simulink subsystem "PvtSubSys_LATC"  (R2020b)
settings: Solver=VariableStepAuto  StartTime=0.0  StopTime=10.0  RelTol=1e-3
undefined symbols (not defined in the file or in its folder): LCS_PLAN_PreViewIdxNum, LCS_PLAN_PreViewIdxSW_b, P_Global_CharSpd_ms, P_Global_SteeringAngleRatio, P_Global_WheelBase_m, P_LCS_DetNoOverRide_DrvTrq_TH, P_LCS_DetOverRide_DrvTrq_TH, P_LCS_ESS_AngleSlope_Limit, P_LCS_ESS_LogicTest_Enable, P_LCS_ESS_NotActiveFlgDelayTime, P_LCS_ESS_NotActiveFlgDelayTimeSW, P_LCS_ESS_SteerAngleErr, P_LCS_ESS_SteerAngleFilterTime, P_LCS_ESS_TarAngleFilterTime, P_LCS_ESSAngleSW, P_LCS_ESSOverrideTime1, P_LCS_ESSOverrideTime2, P_LCS_ESSOverrideTime3, P_LCS_ESSOverrideValue1, P_LCS_ESSOverrideValue2, P_LCS_IN_Offset_Test_SW, P_LCS_IN_Offset_Test_Value, P_LCS_LATC_AngleFilterTime_s, P_LCS_LATC_CurOffsetA2FliterT_s, P_LCS_LATC_CurOffsetCurve_TabX_m, P_LCS_LATC_CurOffsetCurveFliterTime_Tab_s, P_LCS_LATC_CurOffsetVehicleSpdLimitValue_degs, P_LCS_LATC_DeltaEps_Tab_s, P_LCS_LATC_DxOffset_Sw, P_LCS_LATC_ELKAngleSlope_ratio, P_LCS_LATC_ELKMaxLatAcc_ms2, P_LCS_LATC_ESSA0Dis_TabX_m, P_LCS_LATC_ESSAddAngleSlope_Tab_degs, P_LCS_LATC_ESSAESAngleSlope_Tab_degs, P_LCS_LATC_ESSAngleSlope_ratio, P_LCS_LATC_ESSMaxLatAcc_ms2, P_LCS_LATC_LCAngleSlope_ratio, P_LCS_LATC_LCAngleSlope_Tab_degs, P_LCS_LATC_LCCancleMaxLatAcc_ms2, P_LCS_LATC_LCEcoAngleSlope_ratio, P_LCS_LATC_LCEcoAngleSlope_Tab_degs, P_LCS_LATC_LCEcoMaxLatAcc_ms2, P_LCS_LATC_LCKAngleSlope_ratio, P_LCS_LATC_LCKAngleSlope_Tab_degs, P_LCS_LATC_LCKIEAngleSlope_ratio, P_LCS_LATC_LCKIEAngleSlope_Tab_degs, P_LCS_LATC_LCKIEMaxLatAcc_ms2, P_LCS_LATC_LCKMaxLatAcc_ms2, P_LCS_LATC_LCNormalAngleSlope_ratio, P_LCS_LATC_LCNormalAngleSlope_Tab_degs, P_LCS_LATC_LCNormalMaxLatAcc_ms2, P_LCS_LATC_LCSportAngleSlope_ratio, P_LCS_LATC_LCSportAngleSlope_Tab_degs, P_LCS_LATC_LCSportMaxLatAcc_ms2, P_LCS_LATC_LKAAngleSlope_ratio, P_LCS_LATC_LKAAngleSlope_Tab_degs, P_LCS_LATC_LKAMaxLatAcc_ms2, P_LCS_LATC_MatrixQ1_st, P_LCS_LATC_MatrixQ3_st, P_LCS_LATC_MatrixR_st ... (+71)
libraries: simulink x38
(part 6 of 6)

== matlab function PvtSubSys_LATC/LATC/LateralControl/LCS_Angle/Lateral_Control/kinematics_MPC/SteerAngSlopeCalc/MATLAB Function3 ==
  data: delytime input uint16; TarDangerLevel input uint8; TarDangerLevelK1 input uint8; FLg output uint8; FLgK1 input uint8; CntK1 input uint16; Cnt output uint16
function [FLg,Cnt] = AngSlopeCalc(delytime,TarDangerLevel,TarDangerLevelK1,FLgK1,CntK1)

Cnt = min(CntK1 + uint16(1),delytime);
if Cnt== delytime
    FLg = uint8(0);
else
    FLg = FLgK1;
end
%FLg = FLgK1;
%% 
if TarDangerLevel==uint8(1) && TarDangerLevelK1==0  % NO function 2 LCK (TarDangerLevelK1==0)
    Cnt =uint16(0);
    FLg = uint8(1);
end

if  TarDangerLevel==uint8(3) && (TarDangerLevelK1==uint8(1)||TarDangerLevelK1==uint8(2)) % LCK/IE 2 LC_Normal
    Cnt =uint16(0);
    FLg = uint8(2);
end

if  TarDangerLevel==uint8(7) && (TarDangerLevelK1==uint8(1)||TarDangerLevelK1==uint8(2)) % LCK/IE 2 LC_Eco
    Cnt =uint16(0);
    FLg = uint8(3);
end

if  TarDangerLevel==uint8(8) && (TarDangerLevelK1==uint8(1)||TarDangerLevelK1==uint8(2)) % LCK/IE 2 LC_sport
    Cnt =uint16(0);
    FLg = uint8(4);
end
if  TarDangerLevel==uint8(6) && (TarDangerLevelK1==uint8(1)||TarDangerLevelK1==uint8(2)) % LCK/IE 2 ESS 后期添加配和ESS Slope 一起调试
    Cnt =uint16(0);
    FLg = uint8(5);
end

== matlab function PvtSubSys_LATC/LATC/LateralControl/LCS_Angle/Lateral_Control/kinematics_MPC/TarSteerAngleCalc ==
  data: steer_angle_cmd_temp output; steer_feedforward_temp output; steer_feedbackward_temp output; steer_limit_temp output; matrix_result output; LineValid input; SteerAngle input; steer_angle output size=[1,1]; Veh_Speed input; ref_curve input; ref_theta input; Delta_t input; lateral_error input; heading_error input; Umax input; Delta_umax input; Left_steer_ratio input; Right_steer_ratio input; Matrix_q1 input; Matrix_q2 input; Matrix_r input; Max_lateral_acceleration input; TarSteerAngleSlope input; CurrentSteerAngleOffset input; steer_angleK1 input single; U_k output; U_k1 input single
function [steer_angle_cmd_temp,steer_feedforward_temp,steer_feedbackward_temp,steer_limit_temp,matrix_result,steer_angle,U_k]= ...
    kinematics_MPC(LineValid,SteerAngle,Veh_Speed,ref_curve,ref_theta,Delta_t,lateral_error,heading_error,Umax,Delta_umax,...
    Left_steer_ratio,Right_steer_ratio,Matrix_q1,Matrix_q2,Matrix_r,Max_lateral_acceleration,TarSteerAngleSlope,CurrentSteerAngleOffset,steer_angleK1,U_k1)
if LineValid
    %% 1.车辆参数
    %1.1 车的大小及长度参数
    veh_params.vehicle_length = single(4.875);
    veh_params.vehicle_width  = single(2.2);
    veh_params.vehicle_height = single(1.69);
    %1.2 车辆控制参数
    veh_params.wheel_base = single(2.92);               %轴距, m
    veh_params.Vch = single(23.5);                      %特征车速
    veh_params.max_steer_angle = single(53 / 180 * pi); %前轮最大转角  
    veh_params.max_acceleration = single(2);            %车辆最大加速度
    veh_params.max_deceleration = single(-2);           %车辆最大减速度
    veh_params.left_steer_ratio = Left_steer_ratio;     %车辆左侧转向传动比%
    veh_params.right_steer_ratio = Right_steer_ratio;   %车辆右侧转向传动比%
    veh_params.cf = single(155494.663);                 %车辆前轮侧偏刚度
    veh_params.cr = single(155494.663);                 %车辆后轮侧偏刚度 
    veh_params.mass_fl = single(520);                   %车辆左前轮负重
    veh_params.mass_fr = single(520);                   %车辆右前轮负重
    veh_params.mass_rl = single(520);                   %车辆左后轮负重
    veh_params.mass_rr = single(520);                   %车辆右后轮负重
    %% 2.控制参数计算
    %% 3.MPC矩阵
    Np = single(10);
    Nc = single(5);
    Row = single(10); %松弛因子
    ref_delta = atan(veh_params.wheel_base * ref_curve);   %前轮转角
    
    A = [ 1  Veh_Speed * cos(ref_theta) * Delta_t;
          0  1 ];
    B = [ 0;
        Veh_Speed * Delta_t / (veh_params.wheel_base * cos(ref_delta)^2)];
    Nx = size(A,1); %状态量的个数 2
    Nu = size(B,2); %控制量的个数 1
    % 对状态量进行增广
    kesi = zeros(Nx,1); % 构造新的状态量矩阵
    kesi = cat(1,kesi,U_k1);% 将上一时刻的前轮偏角误差放在第3行，进行状态增广3*1维矩阵
    kesi(1) = lateral_error;
    kesi(2) = heading_error;
    %定义Q和R矩阵
    matrix_q = [Matrix_q1 0;
                0 Matrix_q2];
    matrix_r = Matrix_r;
    matrix_Q = zeros(Np*Nx,Np*Nx);%20*20
    matrix_Q_temp = zeros(Nx,Np*Nx);%2*20
    for i=1:Np
        for j= 1:Np
            if i == j
                matrix_Q_temp = zeros(Nx,Np*Nx);
                matrix_Q_temp(:,((j-1)*Nx+1):j*Nx) = matrix_q;
            end
        end
        matrix_Q(((i-1)*Nx+1):i*Nx,:) = matrix_Q_temp;
    end
    matrix_R = zeros(Nc*Nu,Nc*Nu);%10*10
    matrix_R_temp = zeros(Nu,Nc*Nu);
    for i=1:Nc
        for j= 1:Nc
            if i == j
                matrix_R_temp = zeros(Nu,Nc*Nu);
                matrix_R_temp(:,((j-1)*Nu+1):j*Nu) = matrix_r;
            end
        end
        matrix_R(((i-1)*Nu+1):i*Nu,:) = matrix_R_temp;
    end
    % 按增量式对矩阵进行增广
    A = [A B;zeros(Nu,Nx) eye(Nu)]; % 3*3
    B = [B;eye(Nu)]; % 3*1
    % 定义输出矩阵
    C = single([1 0 0;0 1 0;]);% 2*3
    % THETA和PHI
    PHI = zeros(Np*Nx,size(A,2));
    THETA = zeros(Np*Nx,Nc*Nu);
    THETA_temp = zeros(Nx,Nc*Nu);
    for r=1:Np
        for c=1:Nc
            if c<=r
                THETA_temp(:,((c-1)*Nu+1):c*Nu)=C*A^(r-c)*B; %2*3*3*3*1
            end
        end
        THETA(((r-1)*Nx+1):r*Nx,:) = THETA_temp;
        PHI(((r-1)*Nx+1):r*Nx,:) =  C*A^r; %2*3*3*3
    end
    
    % 构造二次规划的H矩阵
    H_temp = THETA'*matrix_Q*THETA + matrix_R;
    % H = zeros((size(H_temp,1)+1),(size(H_temp,2)+1));
    H = [H_temp zeros(Nu*Nc,1);zeros(1,Nu*Nc) Row];
    H = single(2)*H;
    H = (H+H')/single(2);
    % E矩阵
    error = PHI*kesi; %这里的error就是我们所设的E矩阵
    % f矩阵
    f_temp = single(2)*error'* matrix_Q * THETA;
    f = zeros(size(f_temp,1),(size(f_temp,2)+1));
    f(:,1:size(f_temp,2)) = f_temp;
    %% 约束生成区域
    % 不等式约束
    A_t = tril(ones(Nc,Nc),0);
    A_I=kron(A_t,eye(Nu));
    Ut=kron(ones(Nc,1),U_k1);                 %此处的U表示的应该是上一时刻控制量误差（即偏差）组成的矩阵。
    umin = -Umax/single(57.3);                %维数与控制变量的个数相同
    umax = Umax/single(57.3);                 %此处的最大值最小值约束，是对控制量误差的最大最小值进行约束，此处理解的物理意义是在参考转角上下一个范围内进行约束求解
    
    delta_umin =  -Delta_umax/single(57.3)*Delta_t;
    delta_umax =   Delta_umax/single(57.3)*Delta_t;
    Umin=kron(ones(Nc,1),umin);
    Umax=kron(ones(Nc,1),umax);
%     A_cons = [A_I zeros(Nu*Nc,1);-A_I zeros(Nu*Nc,1)];
%     b_cons = [Umax-Ut;-Umin+Ut];
    % 上下限约束
    EM = single(10);
    delta_Umin=kron(ones(Nc,1),delta_umin);
    delta_Umax=kron(ones(Nc,1),delta_umax);
    lb=[delta_Umin;-EM];%（求解方程）状态量下界，包含控制时域内控制增量和松弛因子下界M
    ub=[delta_Umax;EM];%（求解方程）状态量上界，包含控制时域内控制增量和松弛因子上界M
    % 两种约束合并
    A_cons2 = [A_I zeros(Nu*Nc,1);-A_I zeros(Nu*Nc,1);eye((Nu*Nc)+1);-eye((Nu*Nc)+1)];
    b_cons2 = [Umax-Ut;-Umin+Ut;ub;-lb];
    %% 二次规划求解
    % Format in qp_solver
    % min 0.5*x'*H*x + f'*x   subject to:  A*x <= b
    % with respect to:  A * x = b (equality constraint)
    % A*x <= b (inequality constraint)
    % solve QR problem
    % [matrix_result] = mpcCustomSolverCodeGen(single(H),single(f), single(-A_cons2), single(-b_cons2));
    matrix_result = single(zeros(Nc+1,1));
    matrix_result = MPC_Solver_QPhild(H,f',A_cons2,b_cons2);
    %% 4.计算前轮转角
    u_piao = matrix_result(1);
    U_k = single(kesi(3)) + u_piao;
    steer_cmd = ref_delta + U_k;
    %% 反算方向盘转角并转换为角度制
    if (steer_cmd>=0)
        steer_transmission_ratio = veh_params.left_steer_ratio;
    else
        steer_transmission_ratio = veh_params.right_steer_ratio;
    end
    steer_feedforward_temp  = ref_delta * single(57.3) * steer_transmission_ratio;%反算方向盘转角并转换为角度制deg
    steer_feedbackward_temp = U_k * single(57.3) * steer_transmission_ratio;%反算方向盘转角并转换为角度制deg
    steer_angle_cmd = steer_cmd * single(57.3) * steer_transmission_ratio;%反算方向盘转角并转换为角度制deg
    steer_angle_cmd_temp = steer_angle_cmd;%输出算法计算角度作为观测，最终请求角度会补偿转向不足。
    %% 5.限制期望前轮偏角
    % 5.1 根据横向加速度限制前轮转角
    if Veh_Speed < 1
        steer_limit = atan( Max_lateral_acceleration * veh_params.wheel_base /(Veh_Speed *Veh_Speed))* single(57.3) * steer_transmission_ratio; % 高速计算不准确，更改为下面特征车速计算方法
    else
        AckConst = min((single(1)+Veh_Speed*Veh_Speed/(veh_params.Vch*veh_params.Vch))*veh_params.wheel_base/max(single(1),Veh_Speed),single(32767));
        % PsiDtAckRaw = (SteerAngle/steer_transmission_ratio)/AckConst;
        steer_limit = ((Max_lateral_acceleration * AckConst)/Veh_Speed)* single(57.3) * steer_transmission_ratio;
    end
    %     steer_limit = atan( Max_lateral_acceleration * veh_params.wheel_base /(Veh_Speed *Veh_Speed)) * steer_transmission_ratio;
    steer_angle_cmd = min(steer_limit, max(-steer_limit,steer_angle_cmd));%方向盘角度制deg
    
    steer_angle_deg = steer_angle_cmd + CurrentSteerAngleOffset;
    steer_limit_temp = steer_limit;
    % 5.2 限制方向盘转速
    steer_angle = min(steer_angleK1 + TarSteerAngleSlope,max(steer_angleK1 - TarSteerAngleSlope,steer_angle_deg));
    
else
    U_k = single(0);
    matrix_result = single(zeros(6,1));
    steer_angle = SteerAngle;
    steer_angle_cmd_temp = single(0);
    steer_feedforward_temp = single(0);
    steer_feedbackward_temp = single(0);
    steer_limit_temp = single(0);
end
end

== matlab function PvtSubSys_LATC/LATC/LateralControl/LCS_Angle/Lateral_Control/MPC/Understeer_Offset_Calc/YOD_Ackman ==
  data: AckConst output; VxvRef input; Vch input; WheelBase input; AlpWheelAngle input; PsiDtAckK1 input single; PsiDtAck output
function [AckConst,PsiDtAck] = Ackman(VxvRef,Vch,WheelBase,AlpWheelAngle,PsiDtAckK1)
%#codegen
if VxvRef==uint8(0)%转换常数数据类型
    PsiDtAckRaw = single(0);%转换常数数据类型
    AckConst = single(1);%转换常数数据类型
else
    AckConst = min((single(1)+VxvRef*VxvRef/(Vch*Vch))*WheelBase/VxvRef,single(32767));%转换常数数据类型
    PsiDtAckRaw = AlpWheelAngle/AckConst;
end
PsiDtAck = (single(0.02/0.1))*(PsiDtAckRaw-PsiDtAckK1)+PsiDtAckK1;%转换常数数据类型

== matlab function PvtSubSys_LATC/LATC/LateralControl/LCS_Angle/Motion_Planning/FrenetTrajectory_Lateral/Subsystem1/MATLAB Function ==
  data: Forward_PreViewT input; VehSpd input; PreCurve output; C2 input; C3 input; PreCurve_Abs output
function [PreCurve,PreCurve_Abs]= PreView_Point_Curvature(Forward_PreViewT,VehSpd,C2,C3)
LookForwardDis = VehSpd * Forward_PreViewT;
PreCurve = 6*C3*LookForwardDis + 2*C2;
PreCurve_Abs = abs(PreCurve);
end

== matlab function PvtSubSys_LATC/LATC/LateralControl/LCS_Angle/Lateral_Control/MPC/TargetSteerAngleCalc/MATLAB Function ==
  data: c2 input; c1 input; c3 input; v input; PreCurve output; time input
function PreCurve = fcn(c2,c1,c3,v,time)
pdis = v*time;
% y1 = 3*c3*pdis^2 + 2*c2*pdis + c1;
PreCurve = 6*c3*pdis + 2*c2;
% r = y2/power((1+y1*y1),single(1.5));
end

== matlab function PvtSubSys_LATC/LATC/LateralControl/LCS_Angle/Motion_Planning/FrenetTrajectory_Lateral/Subsystem1/MATLAB Function1 ==
  data: Delaytime input uint16; Flg output uint8; Count output uint16; TarDangerLevel input uint8; TarDangerLevelK1 input uint8; FlgK1 input uint8; CountK1 input uint16
function [Flg,Count]= fcn(Delaytime,TarDangerLevel,TarDangerLevelK1,FlgK1,CountK1)
Count = min(CountK1 + uint16(1),Delaytime);
if Count == Delaytime
    Flg = uint8(0);
else
    Flg = FlgK1;
end
%%状态检测
if TarDangerLevel == uint8(1) && TarDangerLevelK1 == 0 %功能激活
    Count = uint16(0);
    Flg = uint8(1);  
end
end

== matlab function PvtSubSys_LATC/LATC/LateralControl/LCS_Angle/Motion_Planning/CartesianTrajectory_MPC/Subsystem/MATLAB Function ==
  data: c2 input; c1 input; c3 input; v input; PreCurve output; time input
function PreCurve = fcn(c2,c1,c3,v,time)
pdis = v*time;
% y1 = 3*c3*pdis^2 + 2*c2*pdis + c1;
PreCurve = 6*c3*pdis + 2*c2;
% r = y2/power((1+y1*y1),single(1.5));
end

== matlab function PvtSubSys_LATC/LATC/LateralControl/LCS_Angle/Lateral_Control/kinematics_MPC/Understeer&Offset_Calc/YOD_Ackman ==
  data: AckConst output; VxvRef input; Vch input; WheelBase input; AlpWheelAngle input; PsiDtAckK1 input single; PsiDtAck output
function [AckConst,PsiDtAck] = Ackman(VxvRef,Vch,WheelBase,AlpWheelAngle,PsiDtAckK1)
%#codegen
if VxvRef==uint8(0)%转换常数数据类型
    PsiDtAckRaw = single(0);%转换常数数据类型
    AckConst = single(1);%转换常数数据类型
else
    AckConst = min((single(1)+VxvRef*VxvRef/(Vch*Vch))*WheelBase/VxvRef,single(32767));%转换常数数据类型
    PsiDtAckRaw = AlpWheelAngle/AckConst;
end
PsiDtAck = (single(0.02/0.1))*(PsiDtAckRaw-PsiDtAckK1)+PsiDtAckK1;%转换常数数据类型

== matlab function PvtSubSys_LATC/LATC/LateralControl/LCS_Angle/Lateral_Control/kinematics_MPC/MATLAB Function ==
  data: PreviewX input; Delta_t output single; PreviewY input; VehSpd input
function Delta_t = fcn(PreviewX,PreviewY,VehSpd)
L = sqrt((PreviewX)^2 + (PreviewY)^2);
Delta_t = L/single(10*VehSpd);
end

== matlab function PvtSubSys_LATC/LATC/LateralControl/LCS_Angle/Lateral_Control/Trajectory_MPC/TargetSteerAngleCalc/MATLAB Function ==
  data: c2 input; c1 input; c3 input; v input; PreCurve output; time input
function PreCurve = fcn(c2,c1,c3,v,time)
pdis = v*time;
% y1 = 3*c3*pdis^2 + 2*c2*pdis + c1;
PreCurve = 6*c3*pdis + 2*c2;
% r = y2/power((1+y1*y1),single(1.5));
end

== matlab function PvtSubSys_LATC/LATC/LateralControl/LCS_Angle/Lateral_Control/Trajectory_MPC/TargetSteerAngleCalc/MATLAB Function3 ==
  data: delytime input uint16; TarDangerLevel input uint8; TarDangerLevelK1 input uint8; FLg output uint8; FLgK1 input uint8; CntK1 input uint16; Cnt output uint16
function [FLg,Cnt] = AngSlopeCalc(delytime,TarDangerLevel,TarDangerLevelK1,FLgK1,CntK1)

Cnt = min(CntK1 + uint16(1),delytime);
if Cnt== delytime
    FLg = uint8(0);
else
    FLg = FLgK1;
end
%FLg = FLgK1;
%% 换道开始检测
if TarDangerLevel==uint8(1) && TarDangerLevelK1==0  % NO function 2 LCK (TarDangerLevelK1==0)
    Cnt =uint16(0);
    FLg = uint8(1);
end
%由LCK状态切换为Normal
if  TarDangerLevel==uint8(3) && (TarDangerLevelK1==uint8(1)||TarDangerLevelK1==uint8(2)) % LCK/IE 2 LC_Normal
    Cnt =uint16(0);
    FLg = uint8(2);
end
%由LCK状态切换为Eco
if  TarDangerLevel==uint8(7) && (TarDangerLevelK1==uint8(1)||TarDangerLevelK1==uint8(2)) % LCK/IE 2 LC_Eco
    Cnt =uint16(0);
    FLg = uint8(3);
end
%由LCK状态切换为Sport
if  TarDangerLevel==uint8(8) && (TarDangerLevelK1==uint8(1)||TarDangerLevelK1==uint8(2)) % LCK/IE 2 LC_sport
    Cnt =uint16(0);
    FLg = uint8(4);
end
if  TarDangerLevel==uint8(6) && (TarDangerLevelK1==uint8(1)||TarDangerLevelK1==uint8(2)) % LCK/IE 2 ESS 后期添加配和ESS Slope 一起调试
    Cnt =uint16(0);
    FLg = uint8(5);
end
%% 换道完成检测，主要时为了解决换道完成后切换到LCK后Angleslope太小导致超调，检测到换道完成后延时一段时间保持一个大斜率。
if  (TarDangerLevel==uint8(1)||TarDangerLevel==uint8(2)) && (TarDangerLevelK1==uint8(3)) % LCK/IE 2 LC_Normal Complete
    Cnt =uint16(0);
    FLg = uint8(6);
end
if  (TarDangerLevel==uint8(1)||TarDangerLevel==uint8(2)) && (TarDangerLevelK1==uint8(7)) % LCK/IE 2 LC_Eco Complete
    Cnt =uint16(0);
    FLg = uint8(7);
end
if  (TarDangerLevel==uint8(1)||TarDangerLevel==uint8(2)) && (TarDangerLevelK1==uint8(8)) % LCK/IE 2 LC_sport Complete
    Cnt =uint16(0);
    FLg = uint8(8);
end

== matlab function PvtSubSys_LATC/LATC/LateralControl/LCS_Angle/Lateral_Control/Trajectory_MPC/TargetSteerAngleCalc/TargetSteerAngleCalc ==
  data: LineValid input boolean size=1; TarSteerAngle output single size=1; TarSteerAngleEnd output single size=1; Xn output single; Yn output single; Yawn output single; Num output uint8 size=1; J output single; Jr1 output single; Jq output single; vxvRef input single size=1; SteerAngle input single size=1; Charspd input single size=1; WheelBase input single size=1; SteerRatio input single size=1; tDeltaEPS input single size=1; PreDis input single size=1; TarSteerAngleSlope input single size=1; R1 input single size=1; Q input single size=1; TarSteerAngleK1 input single size=1; ADDANGLE output; CurrentSteerAngleOffset input single; SteerAngleOffset_deg input; LCS_PlanX input; LCS_PlanY input
function [TarSteerAngle,TarSteerAngleEnd,Xn,Yn,Yawn,Num,J,Jr1,Jq,ADDANGLE] = ...
    TargetSteerAngleCalc(LineValid,vxvRef,SteerAngle,Charspd,WheelBase,SteerRatio,tDeltaEPS,PreDis,TarSteerAngleSlope,R1,Q,...
    TarSteerAngleK1,CurrentSteerAngleOffset,SteerAngleOffset_deg,...
    LCS_PlanX,LCS_PlanY)

StrToWhlFac = 57.3*SteerRatio;  %弧度转换角度
SteerAngleSpdLimit = single(TarSteerAngleSlope*50);  %方向盘转动变化率限制(°/s)
dxOffset = single(2.1);  %车辆前轴的距离

Delta = single([-45,-40, -35, -30,-27,-24,-21, -18,-15, -12,-10, -8,-6,-5,...
         -4.5,-4,-3.5,-3, -2.5,-2, -1.5, -1,-0.5, 0,0.5, 1, 1.5, 2,...
         2.5,3,3.5,4,4.5, 5 ,6 ,8, 10,12,15,18,21,24,27,30,35,40,45]);

J = single(zeros(length(Delta),1));
Jr1 = single(zeros(length(Delta),1));
Jq = single(zeros(length(Delta),1));
vRef = max(vxvRef,single(0.1));

if LineValid
    % 20 Calculate Cycle
    Step_Dis = PreDis/single(49);                   %将规划轨迹均分50等份
    SteerAngleMa = single(zeros(length(Delta),20)); %方向盘转角矩阵
    YawMa = single(zeros(length(Delta),20));        %车身朝向角
    YiMa = single(zeros(length(Delta),20));         %横坐标
    XiMa = single(zeros(length(Delta),20));         %纵坐标
    Traj_Valid = true(length(Delta),1);
    Jmin =single(-1);
    Num = uint8(0);

    for k = uint8(1:1:length(Delta))
        SteerAngleRaw = SteerAngle + Delta(k);       %方向盘实际有效转角+预期方向盘增量
        Step_T = Step_Dis/vRef;                      %行驶完每一份规划轨迹所用的时间（预测步长）
        %% 推算每条轨迹下每个轨迹点处方向盘转角
        SteerAngleMa(k,1) =  TarSteerAngleK1;        %计算31条轨迹起始位置的方向盘转角
        for i = 2:20                                 %每条轨迹的20个轨迹点之间的预测步长选择（变步长）
            if i<=5
                Delta_T = Step_T * single((i-1));
            elseif i<=10
                Delta_T = 4*Step_T + 2*Step_T*single((i-5));
            elseif i<=15
                Delta_T = 14*Step_T + 3*Step_T*single((i-10));
            else
                Delta_T = 29*Step_T + 4*Step_T*single((i-15));
            end
            
            if SteerAngleRaw > TarSteerAngleK1    %判断转向方向  方向盘转角左正右负  
                SteerAngleMa(k,i) = TarSteerAngleK1 + Delta_T*SteerAngleSpdLimit;%计算每条轨迹下的20个方向盘转角
                SteerAngleMa(k,i) = min(SteerAngleMa(k,i),SteerAngleRaw);% 
            else
                SteerAngleMa(k,i) = TarSteerAngleK1 - Delta_T*SteerAngleSpdLimit;
                SteerAngleMa(k,i) = max(SteerAngleMa(k,i),SteerAngleRaw);
            end
        end
        %% 计算每条轨迹起始点(第一个点)的坐标及车身朝向角
        if vRef<1
            YawMa(k,1) = tDeltaEPS*vRef*tan((SteerAngle)/StrToWhlFac)/WheelBase; % 计算每一条推算轨迹起始位置的车身朝向角（单位：rad）
        else
            AckConst = min((single(1)+vRef*vRef/(Charspd*Charspd))*WheelBase/max(single(1),vRef),single(32767));  %计算稳态横摆角速度增益 （单位：s）
            YawMa(k,1) = tDeltaEPS*(SteerAngle)/(AckConst*StrToWhlFac);     % 计算每一条推算轨迹起始位置的车身朝向角(角度)
        end
        XiMa(k,1) = tDeltaEPS*vRef*cos(YawMa(k,1));%推算第一步纵向坐标
        YiMa(k,1) = tDeltaEPS*vRef*sin(YawMa(k,1));%推算第一步横向坐标
        %% 转向cost
        uDelta = SteerAngleMa(k,3) - SteerAngleMa(k,1);
        %%
        for i=1:19
            if i<=5
                StepDisFac = single(1);
            elseif i<=10
                StepDisFac = single(2);
            elseif i<=15
                StepDisFac = single(3);
            else
                StepDisFac = single(4);
            end
            if vRef<1
                t_kap = tan(SteerAngleMa(k,i)/StrToWhlFac)/WheelBase;  %计算每一个方向盘转角下对应的曲率
                YawMa(k,i+1) = YawMa(k,i) + StepDisFac*Step_Dis*t_kap;  %计算每一条推算轨迹除起始位置的车身朝向角
            else
                T_Step = StepDisFac*Step_Dis/vRef;
                AckConst = min((single(1)+vRef*vRef/(Charspd*Charspd))*WheelBase/vRef,single(32767));
                YawRate = SteerAngleMa(k,i)/(AckConst*StrToWhlFac); % 横摆角速度
                YawMa(k,i+1) = YawMa(k,i) + YawRate*T_Step;         % 每一步结束后的车辆朝向角
            end
            
            if (YawMa(k,i+1)>single(1.2))||(YawMa(k,i+1)<single(-1.2)) %筛选推算轨迹(如果朝向角度相对于参考线误差太大直接舍去)
                Traj_Valid(k) = false;
            else
                XiMa(k,i+1) = XiMa(k,i) + StepDisFac*Step_Dis *cos(0.5*(YawMa(k,i)+YawMa(k,i+1))); %计算每一个推算点的纵向坐标 XiMa(k,i+1) = XiMa(k,i) + StepDisFac*Step_Dis *cos((YawMa(k,i));
                YiMa(k,i+1) = YiMa(k,i) + StepDisFac*Step_Dis *sin(0.5*(YawMa(k,i)+YawMa(k,i+1))); %计算每一个推算点的横向坐标
            end
        end
        if Traj_Valid(k) == true
            % 推算车辆前轴中心点的位置坐标
            for i = single(1):single(1):single(20)
                XiMa(k,i) = XiMa(k,i) + dxOffset*cos(YawMa(k,i));
                YiMa(k,i) = YiMa(k,i) + dxOffset*sin(YawMa(k,i));
            end
            % 计算损失量
            PlanYi = single(zeros(1,20));
            PlanYi = interp1(LCS_PlanX',LCS_PlanY',XiMa(k,1:20),'linear');
            Jr1(k) = R1*sum(((YiMa(k,1:20) - PlanYi(1,1:20)).^2));      %规划点与控制点之间的横向误差最小（说明两个轨迹贴合程度较高）
            J(k) = J(k) + Jr1(k);
        end   
        % 第K步的损失量
        Jq(k) = Q*uDelta^2;
        J(k) = J(k) + Jq(k);
        % 筛选出最小损失的轨迹
        if Jmin<0
            Jmin = J(k);
            Num = k;
        else
            if J(k)<=Jmin
                Jmin = J(k);
                Num = k;
            end
        end
    end
    TarSteerAngleEnd = SteerAngle + Delta(Num); %算法算出的最终方向盘转角(应该是当前的还是上一帧的存在模糊点)
    TarSteerAngle = min(TarSteerAngleK1 + TarSteerAngleSlope,max(TarSteerAngleK1 - TarSteerAngleSlope,TarSteerAngleEnd)); % 限制方向盘转速
   
    Xn = XiMa(Num,1:20);
    Yn = YiMa(Num,1:20);
    Yawn = YawMa(Num,1:20);
    ADDANGLE=Delta(Num);
else
    TarSteerAngle = SteerAngle+SteerAngleOffset_deg-CurrentSteerAngleOffset;
    TarSteerAngleEnd = SteerAngle;
    Xn = single(zeros(1,20));
    Yn = single(zeros(1,20));
    Yawn = single(zeros(1,20));
    Num = uint8(0);
    ADDANGLE = single(zeros(1,1));
end
end

== matlab function PvtSubSys_LATC/LATC/LateralControl/LCS_Angle/Lateral_Control/Trajectory_MPC/Understeer_Offset_Calc/YOD_Ackman ==
  data: AckConst output; VxvRef input; Vch input; WheelBase input; AlpWheelAngle input; PsiDtAckK1 input single; PsiDtAck output
function [AckConst,PsiDtAck] = Ackman(VxvRef,Vch,WheelBase,AlpWheelAngle,PsiDtAckK1)
%#codegen
if VxvRef==uint8(0)%转换常数数据类型
    PsiDtAckRaw = single(0);%转换常数数据类型
    AckConst = single(1);%转换常数数据类型
else
    AckConst = min((single(1)+VxvRef*VxvRef/(Vch*Vch))*WheelBase/VxvRef,single(32767));%转换常数数据类型
    PsiDtAckRaw = AlpWheelAngle/AckConst;
end
PsiDtAck = (single(0.02/0.1))*(PsiDtAckRaw-PsiDtAckK1)+PsiDtAckK1;%转换常数数据类型

== matlab function PvtSubSys_LATC/LATC/LateralControl/LCS_Angle/Lateral_Control/MPC/TargetSteerAngleCalc/TargetSteerAngleCalc ==
  data: LineValid input boolean size=1; TarSteerAngle output single size=1; TarSteerAngleEnd output single size=1; Xn output single size=1; Yn output single size=1; Yawn output single size=1; Num output single size=1; J output single size=[31,1]; Jr1 output single size=[31,1]; Jq output single size=[31,1]; vxvRef input single size=1; SteerAngle input single size=1; Charspd input single size=1; WheelBase input single size=1; SteerRatio input single size=1; tDeltaEPS input single size=1; preDis input single size=1; TarSteerAngleSlope input single size=1; R1 input single size=1; Q input single size=1; TarSteerAngleK1 input single size=1; XX output; YY output; t_y output; ADDANGLE output; CurrentSteerAngleOffset input single; SteerAngleOffset_deg input; LCS_PlanX input; LCS_PlanY input; preindex input size=[1 7]; preWeight input size=[1 7]; dxoffset_SW input
function [TarSteerAngle,TarSteerAngleEnd,Xn,Yn,Yawn,Num,J,Jr1,Jq,XX,YY,t_y,ADDANGLE] = ...
    TargetSteerAngleCalc(LineValid,vxvRef,SteerAngle,Charspd,WheelBase,SteerRatio,tDeltaEPS,preDis,TarSteerAngleSlope,R1,Q,...
    TarSteerAngleK1,CurrentSteerAngleOffset,SteerAngleOffset_deg,...
    LCS_PlanX,LCS_PlanY,preindex,preWeight,dxoffset_SW)

StrToWhlFac = 57.3*SteerRatio;  %弧度转换角度
SteerAngleDt = single(TarSteerAngleSlope*50);  %每个周期方向盘转动变化率(°/s)
dxOffset = single(2.1);  %车辆质心位置
J = single(zeros(31,1));
Jr1 = single(zeros(31,1));
Jq = single(zeros(31,1));
Num = single(0); 
XX = single(zeros(1,20));
YY = single(zeros(1,20));
t_y = single(zeros(1,20));
ADDANGLE= 0;

deltaAngle = [-45.5, -34.4, -25.3, -18.0, -12.3, -8.0,...
    -4.9, -2.8, -1.5, -0.8, -0.5, -0.4, -0.3, -0.2, -0.1, ...
    0, 0.1, 0.2, 0.3, 0.4, 0.5, 0.8, 1.5, 2.8,...
    4.9, 8.0, 12.3, 18.0, 25.3, 34.4, 45.5];

vRef = max(vxvRef,single(0.1));

if LineValid
    % 20 Calculate Cycle
    disStep = preDis/single(49);         %将规划轨迹均分50等份
    SteerAngleMa = single(zeros(31,20)); %方向盘转角矩阵
    YawMa = single(zeros(31,20));        %车身朝向角
    YiMa = single(zeros(31,20));         %横坐标
    XiMa = single(zeros(31,20));         %纵坐标
    yValid = true(31,1);
    Jmin =single(-1);
    Num = single(0);

    for k=single(1:31)
        SteerAngleRaw = SteerAngle + deltaAngle(k);  %方向盘实际有效转角+预期方向盘增量
        tD = disStep/vRef;                           %行驶完每一份规划轨迹所用的时间（预测步长）
        %% 推算每条轨迹下每个轨迹点处方向盘转角
        SteerAngleMa(k,1) =  TarSteerAngleK1;        %计算31条轨迹起始位置的方向盘转角
        for i=2:20                                   %每条轨迹的20个轨迹点之间的预测步长选择（变步长）
            if i<=5
                tDelta = tD;
            elseif i<=10
                tDelta = 2*tD;
            elseif i<=15
                tDelta = 3*tD;
            else
                tDelta = 4*tD;
            end
            if SteerAngleRaw>SteerAngle    %判断转向方向  方向盘转角左正右负  
                SteerAngleMa(k,i) = SteerAngleMa(k,1) + tDelta*single((i-1))*SteerAngleDt;%计算每条轨迹下的20个方向盘转角
                SteerAngleMa(k,i) = min(SteerAngleMa(k,i),SteerAngleRaw);% 
            else
                SteerAngleMa(k,i) = SteerAngleMa(k,1) - tDelta*(single(i-1))*SteerAngleDt;
                SteerAngleMa(k,i) = max(SteerAngleMa(k,i),SteerAngleRaw);
            end
        end
        %% 计算每条轨迹下起始点的坐标及车身朝向角
        if vRef<1
            YawMa(k,1) = tDeltaEPS*vRef*tan(0.5*(SteerAngle + TarSteerAngleK1)/StrToWhlFac)/WheelBase; % 计算每一条推算轨迹起始位置的车身朝向角（单位：rad）
        else
            AckConst = min((single(1)+vRef*vRef/(Charspd*Charspd))*WheelBase/max(single(1),vRef),single(32767));          %计算稳态横摆角速度增益 （单位：s）
            YawMa(k,1) = 0.5*tDeltaEPS*(SteerAngle + TarSteerAngleK1)/(AckConst*StrToWhlFac);     % 计算每一条推算轨迹起始位置的车身朝向角(角度)
        end
        XiMa(k,1) = tDeltaEPS*vRef*cos(YawMa(k,1));%推算第一步纵向坐标
        YiMa(k,1) = tDeltaEPS*vRef*sin(YawMa(k,1));%推算第一步横向坐标
        %% 
        uDelta = SteerAngleRaw - SteerAngle;

        % t_Start =single(18);
        t_End = single(19); 
        for i=1:t_End
            if i<=5
                disStepFac = single(1);
            elseif i<=10
                disStepFac = single(2);
            elseif i<=15
                disStepFac = single(3);
            else
                disStepFac = single(4);
            end
            if vRef<1
                t_kap = tan(SteerAngleMa(k,i)/StrToWhlFac)/WheelBase;  %计算每一个方向盘转角下对应的曲率
                YawMa(k,i+1) = YawMa(k,i) + disStepFac*disStep*t_kap;  %计算每一条推算轨迹除起始位置的车身朝向角
            else
                tStep = disStepFac*disStep/vRef;
                AckConst = min((single(1)+vRef*vRef/(Charspd*Charspd))*WheelBase/vRef,single(32767));
                YawRate = SteerAngleMa(k,i)/(AckConst*StrToWhlFac); %前轮转角变化率
                YawMa(k,i+1) = YawMa(k,i) + YawRate*tStep;     %计算每一条推算轨迹除起始位置的前轮转角
            end
            
            if (YawMa(k,i+1)>single(1.2))||(YawMa(k,i+1)<single(-1.2)) %筛选推算轨迹
                yValid(k) = false;
            else
                XiMa(k,i+1) = XiMa(k,i) + disStepFac*disStep *cos(0.5*(YawMa(k,i)+YawMa(k,i+1))); %计算每一个推算点的纵向坐标
                YiMa(k,i+1) = YiMa(k,i) + disStepFac*disStep *sin(0.5*(YawMa(k,i)+YawMa(k,i+1))); %计算每一个推算点的横向坐标
            end
        end
        
        if yValid(k) == true
            % 推算车辆中心点的位置坐标
            if dxoffset_SW == 1
                for i = single(1):single(1):single(20)
                    XiMa(k,i) = XiMa(k,i) + dxOffset*cos(YawMa(k,i));
                    YiMa(k,i) = YiMa(k,i) + dxOffset*sin(YawMa(k,i));
                end
            end
            % 计算损失量
            preXi = XiMa(k,preindex);
            preYi = YiMa(k,preindex);
            PlanYi = interp1(LCS_PlanX',LCS_PlanY',preXi,'linear');
            Jr1(k) = R1*sum(((preYi - PlanYi).^2).*preWeight);      %规划点与控制点之间的横向误差最小（说明两个轨迹贴合程度较高）
            J(k) = J(k) + Jr1(k);
        end
        
        %% 第K步的损失量
        Jq(k) = Q*uDelta^2;
        J(k) = J(k) + Jq(k);
        
        if (yValid(k)==true)
            if Jmin<0
                Jmin = J(k);
                Num = k;
            else
                if k<=16
                    if J(k)<=Jmin
                        Jmin = J(k);
                        Num = k;
                    end
                else
                    if J(k)<Jmin
                        Jmin = J(k);
                        Num = k;
                    end
                end
            end
        end
        
    end
    
    TarSteerAngleEnd = SteerAngle + deltaAngle(Num); 
    TarSteerAngle = min(TarSteerAngleK1 + TarSteerAngleSlope,max(TarSteerAngleK1 - TarSteerAngleSlope,TarSteerAngleEnd));
   
    Xn = XiMa(Num,t_End);
    Yn = YiMa(Num,t_End);
    Yawn = YawMa(Num,t_End);
    XX =  XiMa(Num,:);
    YY =  YiMa(Num,:);
    
    ADDANGLE=deltaAngle(Num);
else
    TarSteerAngle = SteerAngle+SteerAngleOffset_deg-CurrentSteerAngleOffset;
    TarSteerAngleEnd = SteerAngle;
    Xn = single(0);
    Yn = single(0);
    Yawn = single(0);
end
end

== matlab function PvtSubSys_LATC/LATC/LateralControl/LCS_Angle/Lateral_Control/Dynamic_Model_LQR/SteerAngSlopeCalc/MATLAB Function3 ==
  data: delytime input uint16; TarDangerLevel input uint8; TarDangerLevelK1 input uint8; FLg output uint8; FLgK1 input uint8; CntK1 input uint16; Cnt output uint16
function [FLg,Cnt] = AngSlopeCalc(delytime,TarDangerLevel,TarDangerLevelK1,FLgK1,CntK1)

Cnt = min(CntK1 + uint16(1),delytime);
if Cnt== delytime
    FLg = uint8(0);
else
    FLg = FLgK1;
end
%FLg = FLgK1;
%% 
if TarDangerLevel==uint8(1) && TarDangerLevelK1==0  % NO function 2 LCK (TarDangerLevelK1==0)
    Cnt =uint16(0);
    FLg = uint8(1);
end

if  TarDangerLevel==uint8(3) && (TarDangerLevelK1==uint8(1)||TarDangerLevelK1==uint8(2)) % LCK/IE 2 LC_Normal
    Cnt =uint16(0);
    FLg = uint8(2);
end

if  TarDangerLevel==uint8(7) && (TarDangerLevelK1==uint8(1)||TarDangerLevelK1==uint8(2)) % LCK/IE 2 LC_Eco
    Cnt =uint16(0);
    FLg = uint8(3);
end

if  TarDangerLevel==uint8(8) && (TarDangerLevelK1==uint8(1)||TarDangerLevelK1==uint8(2)) % LCK/IE 2 LC_sport
    Cnt =uint16(0);
    FLg = uint8(4);
end
if  TarDangerLevel==uint8(6) && (TarDangerLevelK1==uint8(1)||TarDangerLevelK1==uint8(2)) % LCK/IE 2 ESS 后期添加配和ESS Slope 一起调试
    Cnt =uint16(0);
    FLg = uint8(5);
end

== matlab function PvtSubSys_LATC/LATC/LateralControl/LCS_Angle/Lateral_Control/Dynamic_Model_LQR/Understeer&Offset_Calc/YOD_Ackman ==
  data: AckConst output; VxvRef input; Vch input; WheelBase input; AlpWheelAngle input; PsiDtAckK1 input single; PsiDtAck output
function [AckConst,PsiDtAck] = Ackman(VxvRef,Vch,WheelBase,AlpWheelAngle,PsiDtAckK1)
%#codegen
if VxvRef==uint8(0)%转换常数数据类型
    PsiDtAckRaw = single(0);%转换常数数据类型
    AckConst = single(1);%转换常数数据类型
else
    AckConst = min((single(1)+VxvRef*VxvRef/(Vch*Vch))*WheelBase/VxvRef,single(32767));%转换常数数据类型
    PsiDtAckRaw = AlpWheelAngle/AckConst;
end
PsiDtAck = (single(0.02/0.1))*(PsiDtAckRaw-PsiDtAckK1)+PsiDtAckK1;%转换常数数据类型
